simulink model "Wind_Turbine"  (R2023a)
settings: Solver=ode23t  StartTime=0.0  StopTime=200  MaxStep=0.01  RelTol=1e-4  AbsTol=1e-4  EnableMultiTasking=on
PreLoadFcn:
  | warning off Simulink:Commands:LoadMdlParameterizedLink
PostLoadFcn:
  | warning off Simulink:blocks:MatchingGotoNotFound
  | warning off Simulink:blocks:MatchingFromNotFound
  | warning('off','Simulink:SL_OutputNotConnected');
  | warning off Simulink:Engine:SaveWithParameterizedLinks_Warning
  | warning off Simulink:Engine:SaveWithDisabledLinks_Warning
  | warning('off','Simulink:fixpoint:fxpParameterPrecisionLoss');
  | warning off Simulink:blocks:DTConversionUncessary
  | warning off ne_sli:simulator:input:FilteredInputs
  | warning off MATLAB:nearlySingularMatrix
  | 
  | warning off xPCTarget:modeloptions:StackIncrease
  | warning off xPCTarget:sampleTime:sampleTimeInvariance
  | warning off Simulink:blocks:TDelayFixedBuffer
  | 
  | Setup_WT_Configurations
StartFcn:
  | tic
StopFcn:
  | Elapsed_Sim_Time = toc;
  | disp(['Elapsed time is ' num2str(Elapsed_Sim_Time)]);
undefined symbols (not defined in the file): radps2rpm, sigbuilder_block, WT_Params, X, Y, Z
libraries: sm_lib x6, Wind_Lib x4, fl_lib x4, Yaw_System_Lib x4, nesl_utility x3, Pitch_System_Lib x3, Pitch_Controller_Lib x3, spsGroundLib x2, spsThreePhaseVIMeasurementLib x2, Main_Controller_Lib x2, Geartrain_Lib x2, spsThreePhaseSeriesRLCLoadLib x2
(part 2 of 2)

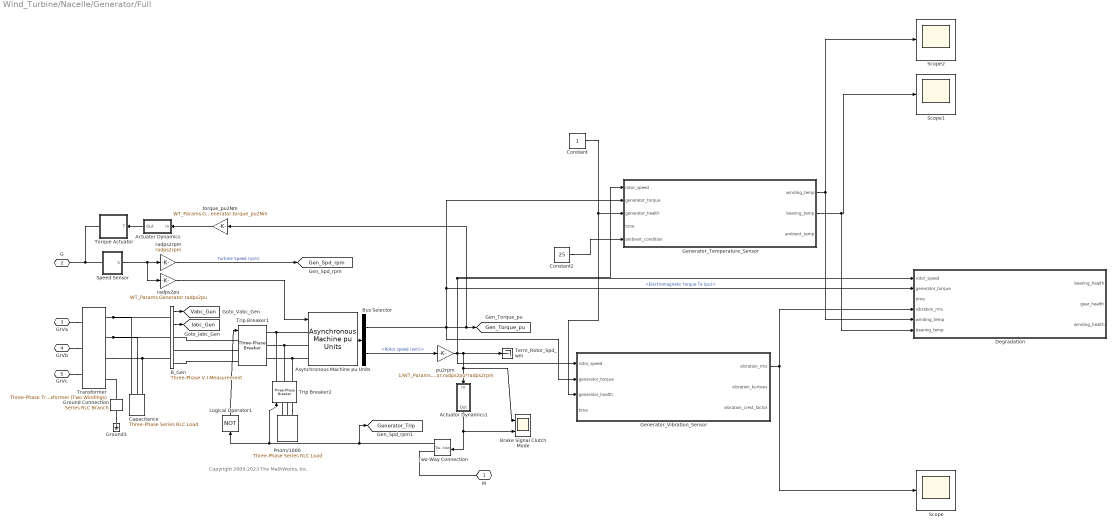
== system Wind_Turbine/Nacelle/Generator/Full ==
  note: Copyright 2009-2023 The MathWorks, Inc.
  Actuator Dynamics : Subsystem  mask(First-order lag supporting vector signals){b=WT_Params.Generator.generator_time_constant, x_initial=0}
      mask prompts: b "Filter time constant"; x_initial "Initial output"
      mask help: Models a lag of the form 1/(b*s+1) where s is the Laplace operator.
  Actuator Dynamics1 : Subsystem  mask(First-order lag supporting vector signals){b=WT_Params.Generator.generator_time_constant, x_initial=0}
      mask prompts: b "Filter time constant"; x_initial "Initial output"
      mask help: Models a lag of the form 1/(b*s+1) where s is the Laplace operator.
  Asynchronous Machine pu Units : spsAsynchronousMachinepuUnitsLib/Asynchronous Machine pu Units  RotorType=Squirrel-cage  PresetModel=No  MechanicalLoad=Speed w  ShowDetailedParameters=on  ReferenceFrame=Rotor  Units=pu  MeasurementBus=off  NominalParameters="[WT_Params.Generator.nominal_power  WT_Params.Generator.voltage WT_Params.Generator.frequency]"  VoltageRatio=1  Stator=[WT_Params.Generator.Stator.resistance WT_Params.Generator.Stator.inductance]  Rotor=[WT_Params.Generator.Rotor.resistance WT_Params.Generator.Rotor.inductance]  Cage1=[0.01909 0.0397]  Cage2=[0.01909 0.0397]  Lm=WT_Params.Generator.mutual_inductance  Mechanical=[0.09526 0.05479 3]  PolePairs=3  InitialConditions=[1 0 0 0 0 0 0 0]  SimulateSaturation=off  Saturation="[0.212,0.4201,0.8125,1.0979,1.4799,2.2457,3.2586,4.5763,6.4763 ;   0.5,0.7,0.9,1,1.1,1.2 ,1.3,1.4,1.5]"  LoadFlowParameters=1650000  TsPowergui=0  TsBlock=-1  IterativeModel=Forward Euler  IterativeDiscreteModel=Trapezoidal non iterative  Pmec=0
  B_Gen : spsThreePhaseVIMeasurementLib/Three-Phase V-I Measurement  VoltageMeasurement=phase-to-ground  SetLabelV=off  LabelV=Vabc  Vpu=on  VpuLL=off  CurrentMeasurement=yes  SetLabelI=off  LabelI=Iabc  Ipu=on  Pbase=WT_Params.Generator.nominal_power  Vbase=WT_Params.Generator.voltage  OutputType=Complex  PhasorSimulation=on  PSBequivalent=0
  Brake Signal Clutch Mode : Scope  NumInputPorts=2
  Bus Selector : BusSelector  OutputSignals=Mechanical.Electromagnetic torque Te (pu),Mechanical.Rotor speed (wm)
  Capacitance : spsThreePhaseSeriesRLCLoadLib/Three-Phase Series RLC Load  LConnTagsString=A|B|C  Configuration=Delta  NominalVoltage=WT_Params.Generator.voltage  Vabc=[1e3 1e3 1e3]  Vabcp=[1e3 1e3 1e3]  NominalFrequency=WT_Params.Generator.frequency  UnbalancedPower=off  ActivePower=0  InductivePower=0  CapacitivePower=200e3  Pabc=[10e3 9e3 11e3]  QLabc=[100 90 110]  QCabc=[100 90 110]  Pabcp=[10e3 9e3 11e3]  QLabcp=[100 90 110]  QCabcp=[100 90 110]  Measurements=None  LoadType=constant Z
  Constant : Constant
  Constant2 : Constant  Value=25
  Degradation : Subsystem
  Generator_Temperature_Sensor : Subsystem
  Generator_Vibration_Sensor : Subsystem
  Ground Connection : spsSeriesRLCBranchLib/Series RLC Branch  LConnTagsString=__new0  RConnTagsString=__new0  BranchType=R  Resistance=10  Inductance=1.0  SetiL0=off  InitialCurrent=0  Capacitance=1.0  Setx0=off  InitialVoltage=0  Measurements=None
  Ground3 : spsGroundLib/Ground  LConnTagsString=a
  Logical Operator1 : Logic  Operator=NOT  AllPortsSameDT=off  OutDataTypeStr=float('double')  SampleTime=0
  Pnom/1000 : spsThreePhaseSeriesRLCLoadLib/Three-Phase Series RLC Load  LConnTagsString=A|B|C  Configuration=Y (grounded)  NominalVoltage=WT_Params.Generator.voltage  Vabc=[1e3 1e3 1e3]  Vabcp=[1e3 1e3 1e3]  NominalFrequency=WT_Params.Generator.frequency  UnbalancedPower=off  ActivePower=WT_Params.Generator.nominal_power  InductivePower=0  CapacitivePower=0  Pabc=[10e3 9e3 11e3]  QLabc=[100 90 110]  QCabc=[100 90 110]  Pabcp=[10e3 9e3 11e3]  QLabcp=[100 90 110]  QCabcp=[100 90 110]  Measurements=None  LoadType=constant Z
  Scope : Scope
  Scope1 : Scope
  Scope2 : Scope
  Speed Sensor : Subsystem
      mask Display:
      | plot([149.600878633536;150.016472378793;150.47508104106;150.972287968219;151.50330478576;152.063017511447;152.646035805762;153.246744883819;153.859359588817;154.477980106257;155.096648782383;155.709407499646;156.310355056631;156.893703999851;157.453836360095;157.985357756531;158.483149347555;158.942417128023;159.358738098149;159.728102859405;160.046954227227;160.312221488639;160.521349974904;160.672325664379;160.763694578642;160.794576785101;160.764674871227;160.674276808796;160.524253180566;160.316048796087;160.051668777399;159.733659248606;159.365082815313;158.949489070056;158.490880407788;157.993673480629;157.462656663088;156.908284800231], [156.971389291536;157.430657072004;157.84697804213;158.216342803387;158.535194171208;158.80046143262;159.009589918885;159.16056560836;159.251934522623;159.282816729083;159.252914815208;159.162516752777;159.012493124547;158.804288740068;158.53990872138;158.221899192587;157.853322759294;157.437729014037;156.979120351769;156.48191342461;155.950896607069;155.391183881382;154.808165587067;154.20745650901;153.594841804012;152.976221286573;152.357552610446;151.744793893183;151.143846336199;150.560497392978;150.000365032735;149.468843636298;148.971052045274;148.511784264806;148.095463294681;147.726098533424;147.407247165603;147.144199990631])
      | plot([152.057635404444;152.93604260309;153.834625296826;154.744729643097;155.657590839533;156.564417533794;157.45647648909;158.325176690034;159.162152078811;159.959342124889;160.709069452336;161.404113777147;162.037781442523;162.603969882449;163.097226392739;163.512800643557;163.846690427691;164.095680203997;164.257372064819;164.330208829146;164.313489039122;164.27939575172], [142.228020686971;141.979030910664;141.817339049842;141.744502285515;141.761222075539;141.867337399197;142.061826307913;142.342815767178;142.707599694895;143.152665022428;143.673725527376;144.265763112236;144.923076131425;145.639334301243;146.40763966397;147.220593018964;148.070365181011;148.948772379657;149.847355073393;150.757459419663;151.6703206161;152.055850472277])
      | plot([116.468514315784;116.438789536125;116.349901463023;116.202706137216;115.998621130155;115.739611892022;115.42817282337;115.067303252679;114.660478551187;114.211616663162;113.725040373958;113.205435679231;112.657806656235;112.087427271827;111.499790591278;110.900555877058;110.29549408704;109.690432297022;109.091197582803;108.503560902254;107.933181517846;107.38555249485;106.865947800123;106.379371510919;105.930509622894;105.523684921402;105.162815350711;104.851376282059;104.592367043926;104.388282036865;104.241086711057;104.152198637956;104.122473858297;104.152198637956;104.241086711057;104.388282036865;104.592367043926;104.851376282059;105.162815350711;105.523684921402;105.930509622894;106.379371510919;106.865947800123;107.38555249485;107.933181517846;108.503560902254;109.091197582803;109.690432297022;110.29549408704;110.900555877058;111.499790591278;112.087427271827;112.657806656235;113.205435679231;113.725040373958;114.211616663162;114.660478551187;115.067303252679;115.42817282337;115.739611892022;115.998621130155;116.202706137216;116.349901463023;116.438789536125;116.468514315784;116.468514315784], [111.618284136057;111.013222346039;110.413987631819;109.826350951271;109.255971566862;108.708342543866;108.188737849139;107.702161559936;107.253299671911;106.846474970419;106.485605399728;106.174166331075;105.915157092943;105.711072085881;105.563876760074;105.474988686973;105.445263907313;105.474988686973;105.563876760074;105.711072085881;105.915157092943;106.174166331075;106.485605399728;106.846474970419;107.253299671911;107.702161559936;108.188737849139;108.708342543866;109.255971566862;109.826350951271;110.413987631819;111.013222346039;111.618284136057;112.223345926075;112.822580640295;113.410217320843;113.980596705252;114.528225728247;115.047830422975;115.534406712178;115.983268600203;116.390093301695;116.750962872386;117.062401941038;117.321411179171;117.525496186232;117.67269151204;117.761579585141;117.7913043648;117.761579585141;117.67269151204;117.525496186232;117.321411179171;117.062401941038;116.750962872386;116.390093301695;115.983268600203;115.534406712178;115.047830422975;114.528225728247;113.980596705252;113.410217320843;112.822580640295;112.223345926075;111.618284136057;111.618284136057])
      | plot([239.23602886498;238.828071429858;237.608127977604;235.587947230552;232.78698463364;229.232214987837;224.957872668068;220.005121927465;214.421660463109;208.261260061133;201.583248745024;194.451939414329;186.936010476274;179.107844435155;171.042830809261;162.818640088593;154.514475725591;146.210311362589;137.986120641921;129.921107016027;122.092940974909;114.577012036853;107.445702706158;100.76769139005;94.607290988073;89.0238295237172;84.0710787831142;79.7967364633452;76.2419668175427;73.4410042206305;71.4208234735788;70.2008800213248;69.7929225862026;70.2008800213248;71.4208234735788;73.4410042206306;76.2419668175428;79.7967364633454;84.0710787831144;89.0238295237174;94.6072909880733;100.76769139005;107.445702706159;114.577012036853;122.092940974909;129.921107016027;137.986120641921;146.210311362589;154.514475725591;162.818640088593;171.042830809261;179.107844435155;186.936010476274;194.451939414329;201.583248745024;208.261260061133;214.421660463109;220.005121927465;224.957872668068;229.232214987837;232.78698463364;235.587947230552;237.608127977604;238.828071429858;239.23602886498;239.23602886498], [155.774275772274;147.47628550917;139.258209428443;131.199192095207;123.376846251889;115.866505365088;108.740498123116;102.067451871182;95.9116316925529;90.3323215006612;85.3832531026163;81.1120887325275;77.5599620381344;74.7610819412943;72.742403187363;71.5233667562631;71.1157126352191;71.5233667562631;72.742403187363;74.7610819412943;77.5599620381345;81.1120887325275;85.3832531026164;90.3323215006612;95.9116316925529;102.067451871182;108.740498123116;115.866505365089;123.376846251889;131.199192095207;139.258209428443;147.47628550917;155.774275772274;164.072266035377;172.290342116104;180.34935944934;188.171705292658;195.682046179459;202.808053421432;209.481099673365;215.636919851994;221.216230043886;226.165298441931;230.43646281202;233.988589506413;236.787469603253;238.806148357184;240.025184788284;240.432838909328;240.025184788284;238.806148357184;236.787469603253;233.988589506413;230.43646281202;226.165298441931;221.216230043886;215.636919851994;209.481099673365;202.808053421432;195.682046179459;188.171705292658;180.34935944934;172.290342116105;164.072266035378;155.774275772274;155.774275772274])
      | plot([252.715889364481;252.243022716633;250.828976737403;248.487369462568;245.240751850236;241.120390602797;236.165967051481;230.425195003451;223.953361231755;216.812793033479;209.072257983804;200.806301666664;192.094529760025;183.020841389688;173.672621134841;164.139897466795;154.514475725591;144.889053984387;135.356330316341;126.008110061494;116.934421691157;108.222649784518;99.9566934673787;92.2161584177032;85.075590219427;78.6037564477313;72.8629843997015;67.9085608483856;63.7881996009461;60.5415819886144;58.199974713779;56.7859287345493;56.3130620867014;56.7859287345493;58.1999747137791;60.5415819886146;63.7881996009463;67.9085608483858;72.8629843997018;78.6037564477315;85.0755902194273;92.2161584177035;99.9566934673791;108.222649784519;116.934421691157;126.008110061494;135.356330316341;144.889053984387;154.514475725591;164.139897466796;173.672621134841;183.020841389688;192.094529760025;200.806301666664;209.072257983803;216.812793033479;223.953361231755;230.425195003451;236.165967051481;241.120390602797;245.240751850236;248.487369462568;250.828976737403;252.243022716633;252.715889364481;252.715889364481], [154.514475725591;144.895228084285;135.36861905618;126.026395093992;116.958526921455;108.252343066071;99.9916888376535;92.2561188521535;85.1201308772245;78.6524483779929;72.9153586725213;67.9641130708855;63.8463947748555;60.6018596625959;58.2617543808809;56.8486154228053;56.3760520890355;56.8486154228053;58.2617543808809;60.6018596625959;63.8463947748555;67.9641130708856;72.9153586725213;78.652448377993;85.1201308772246;92.2561188521536;99.9916888376536;108.252343066072;116.958526921455;126.026395093992;135.36861905618;144.895228084285;154.514475725591;164.133723366898;173.660332395002;183.002556357191;192.070424529728;200.776608385111;209.037262613529;216.772832599029;223.908820573958;230.37650307319;236.113592778661;241.064838380297;245.182556676327;248.427091788587;250.767197070302;252.180336028377;252.652899362147;252.180336028377;250.767197070301;248.427091788587;245.182556676327;241.064838380297;236.113592778661;230.37650307319;223.908820573958;216.772832599029;209.037262613529;200.776608385111;192.070424529728;183.002556357191;173.660332395002;164.133723366898;154.514475725592;154.514475725591])
      | plot([154.514475725591;129.948374815285;179.017586633563;154.514475725591], [240.369848906994;203.583687543869;203.583687543869;240.369848906994])
      | plot([105.382273904979;149.60125554353], [115.271704271436;156.971085816622])
      | plot([144.688035361469;144.688035361469], [152.057865634561;203.583687543869])
      | plot([164.277926087379;164.277926087379], [152.057865634561;203.583687543869])
      | plot([159.112745895982;159.616665914655], [149.60125554353;149.60125554353])
      | plot([115.208714269102;159.364705905318], [107.901873998344;149.60125554353])
      | plot([0;311.800511553884;311.800511553884;0;0], [311.800511553884;311.800511553884;0;0;311.800511553884])
      | ;
      | color('red');
      | port_label('LConn', 1,'R')
      | port_label('output', 1,'W')
  Term_Rotor_Spd_wm : Terminator
  Torque Actuator : Subsystem
      mask Display:
      | plot([198.657636314574;187.5372000791;176.524559560751;165.725772507838;155.244837142898;145.182690602959;135.636236859729;126.697413481378;118.452306223496;110.980319976212;104.353414051689;98.6354091766174;93.8813728637222;90.1370890815176;87.4386173296598;85.811945366254;85.272738931537;85.8261908782356;87.4669711615554;90.1792781704262;93.9369909056548;98.7039205394262;104.434158933498;111.072520759669;118.555074964656;126.809760461083;135.75708011515;145.310866347487;155.379110974044;165.864851295207;176.667103899592;187.681837189509;192.988368326926], [283.691199740558;283.13774779386;281.49696751054;278.784660501669;275.026947766441;270.260018132669;264.529779738597;257.891417912426;250.40886370744;242.154178211013;233.206858556945;223.653072324609;213.584827698051;203.099087376889;192.296834772503;181.282101482586;170.160965409986;159.040529174513;148.027888656163;137.22910160325;126.748166238311;116.686019698372;107.139565955142;98.2007425767901;89.9556353189084;82.4836490716241;75.8567431471018;70.1387382720299;65.3847019591348;61.6404181769301;58.9419464250722;57.3152744616664;56.9214337615639])
      | plot([85.209725657478;1.11807254143059;1.11807254143059], [170.435198815539;170.435198815539;171.380048850551])
      | plot([283.691223012283;397.073227213696], [170.309218810871;170.309218810871])
      | plot([153.301918180659;255.34572196193], [170.309218810871;170.309218810871])
      | plot([198.654719861224;113.618216710165;198.654719861224], [85.2727156598121;170.309218810871;255.34572196193])
      | plot([198.654719861224;153.301918180659;198.654719861224], [215.662020491436;170.309218810871;124.956417130306])
      | plot([198.654719861224;283.691223012283;283.691223012283;187.316519441083;192.985619651154], [283.691223012283;283.691223012283;56.927214609459;56.927214609459;56.927214609459])
      | 
      | patch([395.419739652425;395.419739652425;5.6843418860808e-14;0;395.419739652425;394.947314634919;0.472425017505884;0.472425017505941;394.947314634919;394.947314634919;395.419739652425], [340.618437621742;5.6843418860808e-14;0;340.618437621742;340.618437621742;340.146012604237;340.146012604237;0.472425017505884;0.472425017505884;340.146012604237;340.618437621742], [1;1;1])
      | ;
      | color('red');
      | port_label('RConn', 1,'R')
      | port_label('Input', 1,'T')
  Transformer : spsThreePhaseTransformerTwoWindingsLib/Three-Phase Transformer (Two Windings)  Winding1Connection=Yg  Winding2Connection=Yn  CoreType=Three single-phase transformers  SetSaturation=off  Hysteresis=off  DataFile='hysteresis'  SetInitialFlux=off  Measurements=None  UNITS=pu  NominalPower="[2e6  60]"  Winding1=[WT_Params.Grid.voltage, 0.025/30 , 0.025]  Winding2=[ WT_Params.Generator.voltage, 0.025/30 , 0.025]  Rm=500  Lm=inf  L0=0.5  Saturation=[ 0,0 ; 0.0024,1.2 ; 1.0,1.52 ]  InitialFluxes=[ 0.8 , -0.8 , 0.7 ]  BreakLoop=off  DiscreteSolver=Trapezoidal iterative  DataType=off  TransfoNumber=0
  Trip Breaker1 : spsThreePhaseBreakerLib/Three-Phase Breaker  InitialState=closed  SwitchA=on  SwitchB=on  SwitchC=on  SwitchTimes="[4/60  10/60]"  External=on  BreakerResistance=WT_Params.Generator.Breakers.ron  SnubberResistance=WT_Params.Generator.Breakers.rp  SnubberCapacitance=WT_Params.Generator.Breakers.cp  Measurements=None
  Trip Breaker2 : spsThreePhaseBreakerLib/Three-Phase Breaker  InitialState=open  SwitchA=on  SwitchB=on  SwitchC=on  SwitchTimes="[4/60  10/60]"  External=on  BreakerResistance=WT_Params.Generator.Breakers.ron  SnubberResistance=WT_Params.Generator.Breakers.rp  SnubberCapacitance=WT_Params.Generator.Breakers.cp  Measurements=None
  Two-Way Connection : TwoWayConnection
  pu2rpm : Gain  Gain=1/WT_Params.Generator.radps2pu*radps2rpm
  radps2pu : Gain  Gain=WT_Params.Generator.radps2pu
  radps2rpm : Gain  Gain=radps2rpm
  torque_pu2Nm : Gain  Gain=WT_Params.Generator.torque_pu2Nm
  M : PMIOPort  Tag=PMCPort  Side=Left
  G : PMIOPort  Port=2  Side=Left
  GrVa : PMIOPort  Port=3  Side=Right
  GrVb : PMIOPort  Port=4  Side=Right
  GrVc : PMIOPort  Port=5  Side=Right
  tag scope: Gen_Spd_rpm=global, Gen_Torque_pu=global, Generator_Trip=global, Iabc_Gen=global, Vabc_Gen=global
  wires:
  Actuator Dynamics1/1(Out) -> Two-Way Connection/1, Brake Signal Clutch Mode/2
  Actuator Dynamics/1(Out) -> Torque Actuator/1(T)
  B_Gen/2 -> [Iabc_Gen]
  B_Gen/1 -> [Vabc_Gen]
  Asynchronous Machine pu Units/1 -> Bus Selector/1
  Speed Sensor/1(S) -> radps2rpm/1, radps2pu/1
  Bus Selector/1 -> Generator_Temperature_Sensor/2(generator_torque), Degradation/2(generator_torque), Generator_Vibration_Sensor/2(generator_torque), torque_pu2Nm/1, [Gen_Torque_pu]  "<Electromagnetic torque Te (pu)>"
  radps2pu/1 -> Asynchronous Machine pu Units/1
  torque_pu2Nm/1 -> Actuator Dynamics/1(In)
  radps2rpm/1 -> [Gen_Spd_rpm]  "Turbine Speed (rpm)"
  Bus Selector/2 -> pu2rpm/1  "<Rotor speed (wm)>"
  pu2rpm/1 -> Generator_Temperature_Sensor/1(rotor_speed), Degradation/1(rotor_speed), Generator_Vibration_Sensor/1(rotor_speed), Term_Rotor_Spd_wm/1, Actuator Dynamics1/1(In), Brake Signal Clutch Mode/1
  Two-Way Connection/1 -> [Generator_Trip], Trip Breaker2/1, Logical Operator1/1
  Logical Operator1/1 -> Trip Breaker1/1
  Generator_Vibration_Sensor/1(vibration_rms) -> Scope/1, Degradation/4(vibration_rms)
  Generator_Temperature_Sensor/2(bearing_temp) -> Degradation/6(bearing_temp), Scope1/1
  Generator_Temperature_Sensor/1(winding_temp) -> Degradation/5(winding_temp), Scope2/1
  Constant2/1 -> Generator_Temperature_Sensor/5(ambient_condition)
  Constant/1 -> Generator_Vibration_Sensor/3(generator_health), Generator_Temperature_Sensor/3(generator_health)
  connections:
  Transformer/RConn2 -- B_Gen/LConn2 -- Capacitance/LConn2
  M/RConn1 -- Two-Way Connection/RConn1
  Transformer/RConn1 -- B_Gen/LConn1 -- Capacitance/LConn1
  Transformer/RConn3 -- B_Gen/LConn3 -- Capacitance/LConn3
  Speed Sensor/LConn1 -- G/RConn1 -- Torque Actuator/RConn1
  GrVb/RConn1 -- Transformer/LConn2
  GrVc/RConn1 -- Transformer/LConn3
  GrVa/RConn1 -- Transformer/LConn1
  Ground Connection/RConn1 -- Ground3/LConn1
  Ground Connection/LConn1 -- Transformer/RConn4
  Pnom/1000/LConn1 -- Trip Breaker2/LConn1
  Trip Breaker2/LConn3 -- Pnom/1000/LConn3
  Pnom/1000/LConn2 -- Trip Breaker2/LConn2
  Trip Breaker1/RConn3 -- Asynchronous Machine pu Units/LConn3 -- Trip Breaker2/RConn3
  Trip Breaker1/RConn2 -- Asynchronous Machine pu Units/LConn2 -- Trip Breaker2/RConn2
  Asynchronous Machine pu Units/LConn1 -- Trip Breaker1/RConn1 -- Trip Breaker2/RConn1
  Trip Breaker1/LConn3 -- B_Gen/RConn3
  Trip Breaker1/LConn2 -- B_Gen/RConn2
  Trip Breaker1/LConn1 -- B_Gen/RConn1

== system Wind_Turbine/Scopes/Configure Turbine/Subsystem ==

== system Wind_Turbine/Scopes/Configure Turbine/Subsystem1 ==

== system Wind_Turbine/Scopes/Configure Turbine/Subsystem10 ==

== system Wind_Turbine/Scopes/Configure Turbine/Subsystem11 ==

== system Wind_Turbine/Scopes/Configure Turbine/Subsystem12 ==

== system Wind_Turbine/Scopes/Configure Turbine/Subsystem13 ==

== system Wind_Turbine/Scopes/Configure Turbine/Subsystem14 ==

== system Wind_Turbine/Scopes/Configure Turbine/Subsystem15 ==

== system Wind_Turbine/Scopes/Configure Turbine/Subsystem16 ==

== system Wind_Turbine/Scopes/Configure Turbine/Subsystem17 ==

== system Wind_Turbine/Scopes/Configure Turbine/Subsystem18 ==

== system Wind_Turbine/Scopes/Configure Turbine/Subsystem19 ==

== system Wind_Turbine/Scopes/Configure Turbine/Subsystem2 ==

== system Wind_Turbine/Scopes/Configure Turbine/Subsystem20 ==

== system Wind_Turbine/Scopes/Configure Turbine/Subsystem21 ==

== system Wind_Turbine/Scopes/Configure Turbine/Subsystem22 ==

== system Wind_Turbine/Scopes/Configure Turbine/Subsystem23 ==

== system Wind_Turbine/Scopes/Configure Turbine/Subsystem24 ==

== system Wind_Turbine/Scopes/Configure Turbine/Subsystem3 ==

== system Wind_Turbine/Scopes/Configure Turbine/Subsystem4 ==

== system Wind_Turbine/Scopes/Configure Turbine/Subsystem5 ==

== system Wind_Turbine/Scopes/Configure Turbine/Subsystem6 ==

== system Wind_Turbine/Scopes/Configure Turbine/Subsystem7 ==

== system Wind_Turbine/Scopes/Configure Turbine/Subsystem8 ==

== system Wind_Turbine/Scopes/Configure Turbine/Subsystem9 ==

== system Wind_Turbine/Turbine Input/Commands/Signal Builder ==
  Demux : Demux  Tag=STV Demux  Outputs=1
      settings: DisplayOption=none
  FromWs : FromWorkspace  Tag=STV FromWs  VariableName=tuvar
      SigBuilderData=|
      | common.afterFinalStr = 'Extrapolate'
      | common.sampleTime = 0
      | dataSet(1).timeRange = [0 50]
      | dataSet(1).name = 'Pos_Test'
      | dataSet(2).timeRange = [0 50]
      | dataSet(2).name = 'Pos_Neg_Test'
      | dataSet(3).timeRange = [0 50]
      | dataSet(3).name = 'Step_Test'
      | sbobj.Groups(1).Name = 'Pos_Test'
      | sbobj.Groups(1).Signals.Name = 'Signal 1'
      | sbobj.Groups(1).Signals.XData = [0 5 5 7.5 7.5 25.1 25.1 28 28 50]
      | sbobj.Groups(1).Signals.YData = [0 0 20 20 0 0 20 20 0 0]
      | sbobj.Groups(1).TimeRange = [0 50]
      | sbobj.Groups(2).Name = 'Pos_Neg_Test'
      | sbobj.Groups(2).Signals.Name = 'Signal 1'
      | sbobj.Groups(2).Signals.XData = [0 3 3 5.5 5.5 8 8 10.5 10.5 50]
      | sbobj.Groups(2).Signals.YData = [0 0 20 20 0 0 -20 -20 0 0]
      | sbobj.Groups(2).TimeRange = [0 50]
      | sbobj.Groups(3).Name = 'Step_Test'
      | sbobj.Groups(3).Signals.Name = 'Signal 1'
      | sbobj.Groups(3).Signals.XData = [0 1 1 7.5 25.1 30 30 50]
      | sbobj.Groups(3).Signals.YData = [0 0 20 20 20 20 0 0]
      | sbobj.Groups(3).TimeRange = [0 50]
  Signal 1 : Outport  Tag=STV Outport  VectorParamsAs1DForOutWhenUnconnected=off
  wires:
  Demux/1 -> Signal 1/1
  FromWs/1 -> Demux/1

== system Wind_Turbine/Turbine Input/Commands/Signal Builder2 ==
  Demux : Demux  Tag=STV Demux  Outputs=1
      settings: DisplayOption=none
  FromWs : FromWorkspace  Tag=STV FromWs  VariableName=tuvar
      SigBuilderData=|
      | common.afterFinalStr = 'Extrapolate'
      | common.sampleTime = 0
      | dataSet(1).timeRange = [0 50]
      | dataSet(1).name = 'Pos_Neg_Test'
      | dataSet(2).timeRange = [0 50]
      | dataSet(2).name = 'Step_Test'
      | dataSet(3).timeRange = [0 50]
      | dataSet(3).name = 'Ramp_Test'
      | sbobj.Groups(1).Name = 'Pos_Neg_Test'
      | sbobj.Groups(1).Signals.Name = 'Signal 1'
      | sbobj.Groups(1).Signals.XData = [0 1 1 11 11 21 21 31 31 50]
      | sbobj.Groups(1).Signals.YData = [0 0 4 4 0 0 -4 -4 0 0]
      | sbobj.Groups(2).Name = 'Step_Test'
      | sbobj.Groups(2).Signals.Name = 'Signal 1'
      | sbobj.Groups(2).Signals.XData = [0 1 1 11 21 31 31 50]
      | sbobj.Groups(2).Signals.YData = [0 0 4 4 4 4 0 0]
      | sbobj.Groups(3).Name = 'Ramp_Test'
      | sbobj.Groups(3).Signals.Name = 'Signal 1'
      | sbobj.Groups(3).Signals.XData = [0 1 1 11 21 31 39.1 50]
      | sbobj.Groups(3).Signals.YData = [0 0 2.46 4 2.32 3.18 1.16 0]
  Signal 1 : Outport  Tag=STV Outport  VectorParamsAs1DForOutWhenUnconnected=off
  wires:
  Demux/1 -> Signal 1/1
  FromWs/1 -> Demux/1

== system Wind_Turbine/Turbine Input/Wind/Wind Input ==
  Demux : Demux  Tag=STV Demux  Outputs=2
      settings: DisplayOption=none
  FromWs : FromWorkspace  Tag=STV FromWs  VariableName=tuvar
      SigBuilderData=|
      | common.afterFinalStr = 'Extrapolate'
      | common.sampleTime = 0
      | dataSet(1).timeRange = [0 130]
      | dataSet(1).name = 'Constant Wind No Yaw'
      | dataSet(2).timeRange = [0 130]
      | dataSet(2).name = 'Constant Wind'
      | dataSet(3).timeRange = [0 60]
      | dataSet(3).name = 'High Wind Speed'
      | dataSet(4).timeRange = [0 130]
      | dataSet(4).name = 'Cut Out'
      | dataSet(5).timeRange = [0 130]
      | dataSet(5).name = 'Start Stop'
      | dataSet(6).timeRange = [0 130]
      | dataSet(6).name = 'Start Stop No Yaw'
      | dataSet(7).timeRange = [0 130]
      | dataSet(7).name = 'Varying Wind'
      | sbobj.Groups(1).Name = 'Constant Wind No Yaw'
      | sbobj.Groups(1).Signals(1).Name = 'Wind Speed'
      | sbobj.Groups(1).Signals(1).XData = [0 10 130]
      | sbobj.Groups(1).Signals(1).YData = [10 10 10]
      | sbobj.Groups(1).Signals(2).Name = 'Wind Direction'
      | sbobj.Groups(1).Signals(2).XData = [0 1 11 21 31 130]
      | sbobj.Groups(1).Signals(2).YData = [0 0 0 0 0 0]
      | sbobj.Groups(1).TimeRange = [0 130]
      | sbobj.Groups(2).Name = 'Constant Wind'
      | sbobj.Groups(2).Signals(1).Name = 'Wind Speed'
      | sbobj.Groups(2).Signals(1).XData = [0 10 130]
      | sbobj.Groups(2).Signals(1).YData = [10 10 10]
      | sbobj.Groups(2).Signals(2).Name = 'Wind Direction'
      | sbobj.Groups(2).Signals(2).XData = [0 1 1 11 11 21 21 31 31 130]
      | sbobj.Groups(2).Signals(2).YData = [0 0 4 4 0 0 -4 -4 0 0]
      | sbobj.Groups(2).TimeRange = [0 130]
      | sbobj.Groups(3).Name = 'High Wind Speed'
      | sbobj.Groups(3).Signals(1).Name = 'Wind Speed'
      | sbobj.Groups(3).Signals(1).XData = [0 10 60]
      | sbobj.Groups(3).Signals(1).YData = [10 9.9 25]
      | sbobj.Groups(3).Signals(2).Name = 'Wind Direction'
      | sbobj.Groups(3).Signals(2).XData = [0 1 11 21 31 60]
      | sbobj.Groups(3).Signals(2).YData = [0 0 4 0 -2.1 0]
      | sbobj.Groups(3).TimeRange = [0 60]
      | sbobj.Groups(4).Name = 'Cut Out'
      | sbobj.Groups(4).Signals(1).Name = 'Wind Speed'
      | sbobj.Groups(4).Signals(1).XData = [0 5 25.1 28 60 75 121.8 130]
      | sbobj.Groups(4).Signals(1).YData = [10 10 8.7 7.85 9.65 2 2 2]
      | sbobj.Groups(4).Signals(2).Name = 'Wind Direction'
      | sbobj.Groups(4).Signals(2).XData = [0 1 1 11 11 21 21 31 31 130]
      | sbobj.Groups(4).Signals(2).YData = [0 0 4 4 0 0 -4 -4 0 0]
      | sbobj.Groups(4).TimeRange = [0 130]
      | sbobj.Groups(5).Name = 'Start Stop'
      | sbobj.Groups(5).Signals(1).Name = 'Wind Speed'
      | sbobj.Groups(5).Signals(1).XData = [0 5 25 28 55 75 80 130]
      | sbobj.Groups(5).Signals(1).YData = [2 2 13 10 15 14.9 11.2 11.2]
      | sbobj.Groups(5).Signals(2).Name = 'Wind Direction'
      | sbobj.Groups(5).Signals(2).XData = [0 1 11 21 31 36.6 54.8 75 130]
      | sbobj.Groups(5).Signals(2).YData = [0 0 2.9 0.5 0.5 1.57171717172 0.1 -2.75 -2.85]
      | sbobj.Groups(5).TimeRange = [0 130]
      | sbobj.Groups(6).Name = 'Start Stop No Yaw'
      | sbobj.Groups(6).Signals(1).Name = 'Wind Speed'
      | sbobj.Groups(6).Signals(1).XData = [0 5 25 28 55 75 80 130]
      | sbobj.Groups(6).Signals(1).YData = [2 2 13 10 15 2 2 2]
      | sbobj.Groups(6).Signals(2).Name = 'Wind Direction'
      | sbobj.Groups(6).Signals(2).XData = [0 130]
      | sbobj.Groups(6).Signals(2).YData = [0 0]
      | sbobj.Groups(6).TimeRange = [0 130]
      | sbobj.Groups(7).Name = 'Varying Wind'
      | sbobj.Groups(7).Signals(1).Name = 'Wind Speed'
      | sbobj.Groups(7).Signals(1).XData = [0 5 25 28 45 60.2 75 78.2 80 130]
      | sbobj.Groups(7).Signals(1).YData = [2 2 13 10 14.4 10.6 13.9 8 8 2]
      | sbobj.Groups(7).Signals(2).Name = 'Wind Direction'
      | sbobj.Groups(7).Signals(2).XData = [0 1 11 21 31 36.6 54.8 75 130]
      | sbobj.Groups(7).Signals(2).YData = [0 0 2.9 0.5 0.5 1.57171717172 -4 -4 -4]
      | sbobj.Groups(7).TimeRange = [0 130]
  Wind Speed : Outport  Tag=STV Outport  VectorParamsAs1DForOutWhenUnconnected=off
  Wind Direction : Outport  Tag=STV Outport  Port=2  VectorParamsAs1DForOutWhenUnconnected=off
  wires:
  Demux/2 -> Wind Direction/1
  Demux/1 -> Wind Speed/1
  FromWs/1 -> Demux/1

== system Wind_Turbine/Nacelle/Generator/Full/Actuator Dynamics ==
  In : Inport
  Gain : Gain  Gain=1/b
  Integrator : Integrator  InitialCondition=x_initial
  Sum : Sum  Inputs=|+-  InputSameDT=on  SaturateOnIntegerOverflow=on  OutDataTypeStr=Inherit: Same as first input
  Out : Outport  VectorParamsAs1DForOutWhenUnconnected=off
  wires:
  Sum/1 -> Integrator/1
  In/1 -> Sum/1
  Integrator/1 -> Gain/1
  Gain/1 -> Sum/2, Out/1

== system Wind_Turbine/Nacelle/Generator/Full/Actuator Dynamics1 ==
  In : Inport
  Gain : Gain  Gain=1/b
  Integrator : Integrator  InitialCondition=x_initial
  Sum : Sum  Inputs=|+-  InputSameDT=on  SaturateOnIntegerOverflow=on  OutDataTypeStr=Inherit: Same as first input
  Out : Outport  VectorParamsAs1DForOutWhenUnconnected=off
  wires:
  Gain/1 -> Out/1, Sum/2
  Integrator/1 -> Gain/1
  In/1 -> Sum/1
  Sum/1 -> Integrator/1

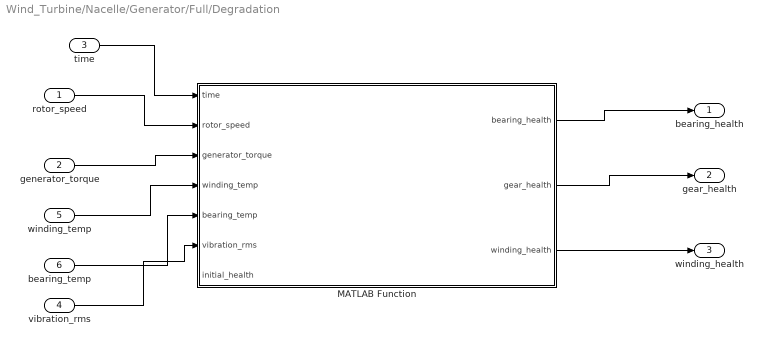
== system Wind_Turbine/Nacelle/Generator/Full/Degradation ==
  rotor_speed : Inport
  generator_torque : Inport  Port=2
  time : Inport  Port=3
  vibration_rms : Inport  Port=4
  winding_temp : Inport  Port=5
  bearing_temp : Inport  Port=6
  MATLAB Function : MATLAB Function  TreatAsAtomicUnit=on
  bearing_health : Outport
  gear_health : Outport  Port=2
  winding_health : Outport  Port=3
  wires:
  rotor_speed/1 -> MATLAB Function/2(rotor_speed)
  generator_torque/1 -> MATLAB Function/3(generator_torque)
  time/1 -> MATLAB Function/1(time)
  MATLAB Function/1(bearing_health) -> bearing_health/1
  MATLAB Function/2(gear_health) -> gear_health/1
  MATLAB Function/3(winding_health) -> winding_health/1
  vibration_rms/1 -> MATLAB Function/6(vibration_rms)
  winding_temp/1 -> MATLAB Function/4(winding_temp)
  bearing_temp/1 -> MATLAB Function/5(bearing_temp)

== system Wind_Turbine/Nacelle/Generator/Full/Generator_Temperature_Sensor ==
  rotor_speed : Inport
  generator_torque : Inport  Port=2
  generator_health : Inport  Port=3
  time : Inport  Port=4
  ambient_condition : Inport  Port=5
  MATLAB Function : MATLAB Function  TreatAsAtomicUnit=on
  winding_temp : Outport
  bearing_temp : Outport  Port=2
  ambient_temp : Outport  Port=3
  wires:
  rotor_speed/1 -> MATLAB Function/1(rotor_speed)
  generator_torque/1 -> MATLAB Function/2(generator_torque)
  generator_health/1 -> MATLAB Function/3(generator_health)
  time/1 -> MATLAB Function/5(time)
  MATLAB Function/1(winding_temp) -> winding_temp/1
  MATLAB Function/2(bearing_temp) -> bearing_temp/1
  MATLAB Function/3(ambient_temp) -> ambient_temp/1
  ambient_condition/1 -> MATLAB Function/4(ambient_condition)

== system Wind_Turbine/Nacelle/Generator/Full/Generator_Vibration_Sensor ==
  rotor_speed : Inport
  generator_torque : Inport  Port=2
  generator_health : Inport  Port=3
  time : Inport  Port=4
  MATLAB Function : MATLAB Function  TreatAsAtomicUnit=on
  vibration_rms : Outport
  vibration_kurtosis : Outport  Port=2
  vibration_crest_factor : Outport  Port=3
  wires:
  rotor_speed/1 -> MATLAB Function/1(rotor_speed)
  generator_torque/1 -> MATLAB Function/2(generator_torque)
  generator_health/1 -> MATLAB Function/3(unused)
  time/1 -> MATLAB Function/4(unused1)
  MATLAB Function/1(vibration_rms) -> vibration_rms/1
  MATLAB Function/2(vibration_kurtosis) -> vibration_kurtosis/1
  MATLAB Function/3(vibration_crest_factor) -> vibration_crest_factor/1

== system Wind_Turbine/Nacelle/Generator/Full/Speed Sensor ==
  Ideal Rotational Motion Sensor : fl_lib/Mechanical/Mechanical Sensors/Ideal Rotational Motion Sensor  reference=foundation.enum.MeasurementReference.difference  acceleration_port=false  velocity_port=true  position_port=true  wrap_angle=simscape.enum.onoff.off  offset=0 rad
  Mechanical Rotational Reference1 : fl_lib/Mechanical/Rotational Elements/Mechanical Rotational Reference
  PS-Simulink Converter : nesl_utility/PS-Simulink Converter  PhysicalDomain=network_engine_domain  SubClassName=ps_output  LeftPortType=input  RightPortType=output  PseudoPeriodic=off  Frequencies=[]  VectorFormat=1-D array  Unit=rad/s  AffineConversion=off
  R : PMIOPort  Side=Left
  S : Outport  VectorParamsAs1DForOutWhenUnconnected=off
  wires:
  PS-Simulink Converter/1 -> S/1
  connections:
  Mechanical Rotational Reference1/LConn1 -- Ideal Rotational Motion Sensor/RConn1
  R/RConn1 -- Ideal Rotational Motion Sensor/LConn1
  Ideal Rotational Motion Sensor/RConn2 -- PS-Simulink Converter/LConn1

== system Wind_Turbine/Nacelle/Generator/Full/Torque Actuator ==
  T : Inport
  Ideal Torque Source : fl_lib/Mechanical/Mechanical Sources/Ideal Torque Source
  Mechanical Rotational Reference : fl_lib/Mechanical/Rotational Elements/Mechanical Rotational Reference
  Simulink-PS Converter : nesl_utility/Simulink-PS Converter  PhysicalDomain=network_engine_domain  SubClassName=ps_input  LeftPortType=input  RightPortType=output  PseudoPeriodic=off  Frequencies=[]  NoiseDistribution=none  NoiseParameters=[]  Unit=1  AffineConversion=off  FilteringAndDerivatives=filter  SimscapeFilterOrder=1  InputFilterTimeConstant=0.005  UdotUserProvided=1
  R : PMIOPort  Side=Right
  wires:
  T/1 -> Simulink-PS Converter/1
  connections:
  R/RConn1 -- Ideal Torque Source/LConn1
  Mechanical Rotational Reference/LConn1 -- Ideal Torque Source/RConn2
  Simulink-PS Converter/RConn1 -- Ideal Torque Source/RConn1

== matlab function Wind_Turbine/Nacelle/Generator/Full/Generator_Temperature_Sensor/MATLAB Function ==
  settings: updateMethod=DISCRETE
  data: rotor_speed input; winding_temp output; generator_torque input; generator_health input; ambient_condition input; bearing_temp output; ambient_temp output; time input
function [winding_temp, bearing_temp, ambient_temp] = generator_temperature_sensor(rotor_speed, generator_torque, generator_health, ambient_condition, time)
    % Generator Temperature Sensor Model
    % Simulates thermal characteristics of a wind turbine generator
    
    % Input parameters:
    % rotor_speed       - RPM of the generator rotor
    % generator_torque  - Torque output (or load) of the generator
    % generator_health  - Health factor (0 to 1, where 1 is perfect health)
    % ambient_condition - Ambient temperature in Celsius
    % time              - Simulation time
    
    % Output parameters:
    % winding_temp      - Temperature of generator windings (°C)
    % bearing_temp      - Temperature of generator bearings (°C)
    % ambient_temp      - Ambient temperature with variations (°C)
    
    % Constants and parameters
    base_winding_temp = 40;    % Base winding temperature at idle (°C)
    base_bearing_temp = 30;    % Base bearing temperature at idle (°C)
    max_winding_temp = 130;    % Maximum winding temperature for healthy generator (°C)
    max_bearing_temp = 90;     % Maximum bearing temperature for healthy generator (°C)
    
    % Thermal coefficients
    winding_thermal_coeff = 0.3;  % How quickly windings heat up with load
    bearing_thermal_coeff = 0.2;  % How quickly bearings heat up with speed
    
    % Safety checks for inputs
    rotor_speed = max(0, abs(rotor_speed));         % Ensure positive speed
    generator_torque = max(0, abs(generator_torque));  % Ensure positive torque
    generator_health = max(0.5, min(1, generator_health));  % Clamp health between 0.5 and 1
    
    % Set default ambient temperature if not provided
    if nargin < 4 || isempty(ambient_condition)
        ambient_condition = 25;  % Default ambient temperature (°C)
    end
    
    % Calculate ambient temperature with minor variations
    ambient_temp = ambient_condition + 2 * sin(0.01 * time);
    
    % Calculate thermal rise due to load and speed
    torque_factor = generator_torque / 100;  % Normalize torque (adjust divisor as needed)
    speed_factor = rotor_speed / 1800;       % Normalize speed (adjust divisor as needed)
    
    % Calculate winding temperature
    winding_rise = winding_thermal_coeff * (torque_factor^2) * (speed_factor) * 100;
    winding_temp = base_winding_temp + winding_rise;
    
    % Add effect of generator health on winding temperature
    % Less healthy generator = more inefficient = more heat
    health_factor_winding = 1 / generator_health;
    winding_temp = winding_temp * health_factor_winding;
    
    % Calculate bearing temperature
    bearing_rise = bearing_thermal_coeff * (speed_factor^1.5) * (torque_factor) * 60;
    bearing_temp = base_bearing_temp + bearing_rise;
    
    % Add effect of generator health on bearing temperature
    health_factor_bearing = 1 / (generator_health^1.5);  % More sensitive to health
    bearing_temp = bearing_temp * health_factor_bearing;
    
    % Limit temperatures to realistic maximum values
    winding_temp = min(winding_temp, 180);  % Absolute maximum 
    bearing_temp = min(bearing_temp, 130);  % Absolute maximum
    
    % Add minor noise to temperature readings (sensor noise)
    rng(round(time*10));  % Seed for reproducible but varying noise
    winding_temp = winding_temp + 0.2 * randn();
    bearing_temp = bearing_temp + 0.1 * randn();
    ambient_temp = ambient_temp + 0.05 * randn();
end

== matlab function Wind_Turbine/Nacelle/Generator/Full/Generator_Vibration_Sensor/MATLAB Function ==
  settings: updateMethod=DISCRETE
  data: rotor_speed input; vibration_rms output; generator_torque input; unused input; unused1 input; vibration_kurtosis output; vibration_crest_factor output
function [vibration_rms, vibration_kurtosis, vibration_crest_factor] = generator_vibration_sensor(rotor_speed, generator_torque, ~, ~)
    % Revised Generator Vibration Sensor Model without degradation
    % Avoids domain errors and other numerical issues
    
    % Parameters
    nominal_speed = 1800;         % rpm (adjust to your generator specs)
    fs = 1000;                    % Sampling frequency (Hz)
    base_amplitude = 0.5;         % mm/s for a healthy generator
    bearing_freq_factor = 0.1;    % Bearing characteristic frequency ratio
    mesh_freq_factor = 8.2;       % Gearmesh frequency multiplier
    
    % Safety check for inputs
    rotor_speed = max(1, abs(rotor_speed));         % Ensure positive non-zero speed
    generator_torque = abs(generator_torque);       % Ensure positive torque
    
    % Calculate rotational frequency in Hz
    freq_rot = rotor_speed / 60;  % convert rpm to Hz
    
    % Load factor using safer formulas (removed health factor)
    load_factor = 1.0 + 0.5 * (generator_torque);    % Linear relationship with torque
    
    % Generate time vector for vibration signal (fixed length regardless of sim time)
    t = 0:(1/fs):(0.1-(1/fs));  % 0.1 second window
    
    % Create empty signal array
    signal = zeros(size(t));
    
    % Add base rotational component
    signal = signal + base_amplitude * sin(2*pi*freq_rot*t);
    
    % Add harmonics
    signal = signal + 0.3 * base_amplitude * sin(2*pi*2*freq_rot*t);  % 2x
    signal = signal + 0.15 * base_amplitude * sin(2*pi*3*freq_rot*t); % 3x
    
    % Add bearing frequencies
    bearing_freq = freq_rot * bearing_freq_factor;
    signal = signal + 0.1 * base_amplitude * sin(2*pi*bearing_freq*t);
    
    % Add gearmesh frequency
    mesh_freq = freq_rot * mesh_freq_factor;
    signal = signal + 0.2 * base_amplitude * sin(2*pi*mesh_freq*t);
    
    % Add random noise
    noise_level = 0.05 * base_amplitude;
    % Use a fixed random seed for reproducibility
    signal = signal + noise_level * randn(size(t));
    
    % Scale by load factor only (removed health factor)
    signal = signal * load_factor;
    
    % Removed fault signatures section that was based on health
    
    % Calculate output metrics (with safety checks)
    % RMS - root mean square (overall vibration energy)
    vibration_rms = sqrt(mean(signal.^2));
    
    % Kurtosis - sensitivity to peaks
    vibration_kurtosis = safe_kurtosis(signal);
    
    % Crest Factor - peak-to-RMS ratio
    peak_value = max(abs(signal));
    if vibration_rms > 0
        vibration_crest_factor = peak_value / vibration_rms;
    else
        vibration_crest_factor = 1.0;  % Default if RMS is zero
    end
end

% Safer version of kurtosis calculation
function k = safe_kurtosis(x)
    n = length(x);
    if n < 4
        % Not enough data points
        k = 3.0;  % Return Gaussian kurtosis
        return;
    end
    
    x_mean = mean(x);
    diff = x - x_mean;
    m2 = mean(diff.^2);  % Second moment (variance)
    
    if m2 < 1e-10
        % Variance too small, avoid division by near-zero
        k = 3.0;  % Return Gaussian kurtosis
    else
        m4 = mean(diff.^4);  % Fourth moment
        k = m4 / (m2^2);     % Kurtosis
    end
end

== matlab function Wind_Turbine/Nacelle/Generator/Full/Degradation/MATLAB Function ==
  settings: updateMethod=DISCRETE
  data: time input; rotor_speed input; bearing_health output; generator_torque input; winding_temp input; bearing_temp input; vibration_rms input; gear_health output; winding_health output; initial_health input
function [bearing_health, gear_health, winding_health] = generator_degradation_model(time, rotor_speed, generator_torque, winding_temp, bearing_temp, vibration_rms, initial_health)
    % Wind Turbine Generator Component Degradation Model
    %
    % Inputs:
    % time             - Simulation time [hours]
    % rotor_speed      - Generator rotor speed [rpm]
    % generator_torque - Generator torque [Nm]
    % winding_temp     - Winding temperature [°C]
    % bearing_temp     - Bearing temperature [°C]
    % vibration_rms    - Vibration RMS value [mm/s]
    % initial_health   - Structure with initial health values for components
    %
    % Outputs:
    % bearing_health   - Remaining useful life percentage of bearings [0-1]
    % gear_health      - Remaining useful life percentage of gears [0-1]
    % winding_health   - Remaining useful life percentage of windings [0-1]
    
    % Parameters for degradation models
    
    % Bearing parameters
    bearing_base_life = 100000;     % Base life in hours (L10 life)
    bearing_temp_threshold = 70;    % Temperature threshold [°C]
    bearing_speed_rated = 1800;     % Rated speed [rpm]
    bearing_load_rated = 100;       % Rated load [Nm]
    
    % Gear parameters
    gear_base_life = 150000;        % Base life in hours
    gear_temp_threshold = 65;       % Temperature threshold [°C]
    gear_vibration_threshold = 5;   % Vibration threshold [mm/s]
    
    % Winding parameters
    winding_base_life = 175000;     % Base life in hours
    winding_temp_threshold = 100;   % Temperature threshold [°C]
    insulation_class_temp = 155;    % Class F insulation max temp [°C]
    
    % Time step calculation (for incremental degradation)
    persistent prev_time;
    if isempty(prev_time)
        prev_time = 0;
    end
    dt = time - prev_time;          % Time difference [hours]
    prev_time = time;
    
    % Persistent variables to track health with proper initialization
    persistent current_bearing_health current_gear_health current_winding_health;
    if isempty(current_bearing_health)
        if nargin >= 7 && isstruct(initial_health)
            % Initialize with provided values if available
            if isfield(initial_health, 'bearing')
                current_bearing_health = initial_health.bearing;
            else
                current_bearing_health = 1.0;
            end
            
            if isfield(initial_health, 'gear')
                current_gear_health = initial_health.gear;
            else
                current_gear_health = 1.0;
            end
            
            if isfield(initial_health, 'winding')
                current_winding_health = initial_health.winding;
            else
                current_winding_health = 1.0;
            end
        else
            % Default initialization
            current_bearing_health = 1.0;
            current_gear_health = 1.0;
            current_winding_health = 1.0;
        end
    end
    
    % Skip degradation if time hasn't advanced
    if dt <= 0
        bearing_health = current_bearing_health;
        gear_health = current_gear_health;
        winding_health = current_winding_health;
        return;
    end
    
    %% Bearing Degradation Model
    % Based on modified L10 life calculation with temperature effects
    
    % Speed and load factors
    speed_factor = max(0.1, min(1.5, rotor_speed / bearing_speed_rated));
    load_factor = max(0.1, min(1.5, generator_torque / bearing_load_rated));
    
    % Basic L10 life calculation (proportional to (load/rated_load)^-3)
    bearing_base_degradation_rate = (load_factor^3) / bearing_base_life;
    
    % Temperature acceleration factor (Arrhenius relationship)
    if bearing_temp > bearing_temp_threshold
        temp_delta = bearing_temp - bearing_temp_threshold;
        bearing_temp_factor = 1.0 + 0.15 * temp_delta; % 15% acceleration per °C above threshold
    else
        bearing_temp_factor = 1.0;
    end
    
    % Vibration effect factor
    vibration_factor = 1.0 + 0.2 * max(0, vibration_rms - 3);
    
    % Combined bearing degradation rate
    bearing_degradation_rate = bearing_base_degradation_rate * bearing_temp_factor * vibration_factor * speed_factor;
    
    % Update bearing health
    bearing_degradation = bearing_degradation_rate * dt;
    current_bearing_health = max(0, current_bearing_health - bearing_degradation);
    
    %% Gear Degradation Model
    % Based on fatigue, wear and temperature effects
    
    % Base degradation rate from load cycling
    gear_load_factor = (load_factor^2.5) / gear_base_life;  
    
    % Temperature effect
    if bearing_temp > gear_temp_threshold
        temp_excess = bearing_temp - gear_temp_threshold;
        gear_temp_factor = 1.0 + 0.1 * temp_excess;  % 10% acceleration per °C above threshold
    else
        gear_temp_factor = 1.0;
    end
    
    % Vibration effect (meshing issues)
    if vibration_rms > gear_vibration_threshold
        gear_vibration_factor = 1.0 + 0.25 * (vibration_rms - gear_vibration_threshold);
    else
        gear_vibration_factor = 1.0;
    end
    
    % Speed variability effect (higher for variable speeds)
    gear_speed_factor = 1.0 + 0.05 * speed_factor;
    
    % Combined gear degradation rate
    gear_degradation_rate = gear_load_factor * gear_temp_factor * gear_vibration_factor * gear_speed_factor;
    
    % Update gear health
    gear_degradation = gear_degradation_rate * dt;
    current_gear_health = max(0, current_gear_health - gear_degradation);
    
    %% Winding Degradation Model
    % Based on insulation degradation following thermal aging (Arrhenius model)
    
    % Base winding degradation rate 
    winding_base_degradation_rate = 1.0 / winding_base_life;
    
    % Temperature effect using exponential thermal aging model
    if winding_temp > winding_temp_threshold
        % Every 10°C increase doubles the aging rate (Montsinger's rule)
        temp_aging_factor = 2^((winding_temp - winding_temp_threshold) / 10);
    else
        temp_aging_factor = 1.0;
    end
    
    % Factor for excessive temperature (approaching insulation class limit)
    if winding_temp > (insulation_class_temp - 20)
        excess_temp_factor = 1.0 + 0.5 * ((winding_temp - (insulation_class_temp - 20)) / 20);
    else
        excess_temp_factor = 1.0;
    end
    
    % Load cycling effect (thermal expansion/contraction stress)
    load_cycling_factor = 1.0 + 0.1 * load_factor;
    
    % Combined winding degradation rate
    winding_degradation_rate = winding_base_degradation_rate * temp_aging_factor * excess_temp_factor * load_cycling_factor;
    
    % Update winding health
    winding_degradation = winding_degradation_rate * dt;
    current_winding_health = max(0, current_winding_health - winding_degradation);
    
    % Return current health values
    bearing_health = current_bearing_health;
    gear_health = current_gear_health;
    winding_health = current_winding_health;
end
